simulink model "BLDC_motor_control_v1"  (R2017b)
settings: Solver=FixedStepDiscrete  StartTime=0.0  StopTime=10  FixedStep=1e-5  RelTol=1e-3
values from neighbouring files (symbols this model uses):
  p = 2    [BLDC_model_init.m]
libraries: nesl_utility x41, fl_lib x33, pe_lib x30, simulink x6, pePwmGenerator x2
(part 2 of 2)

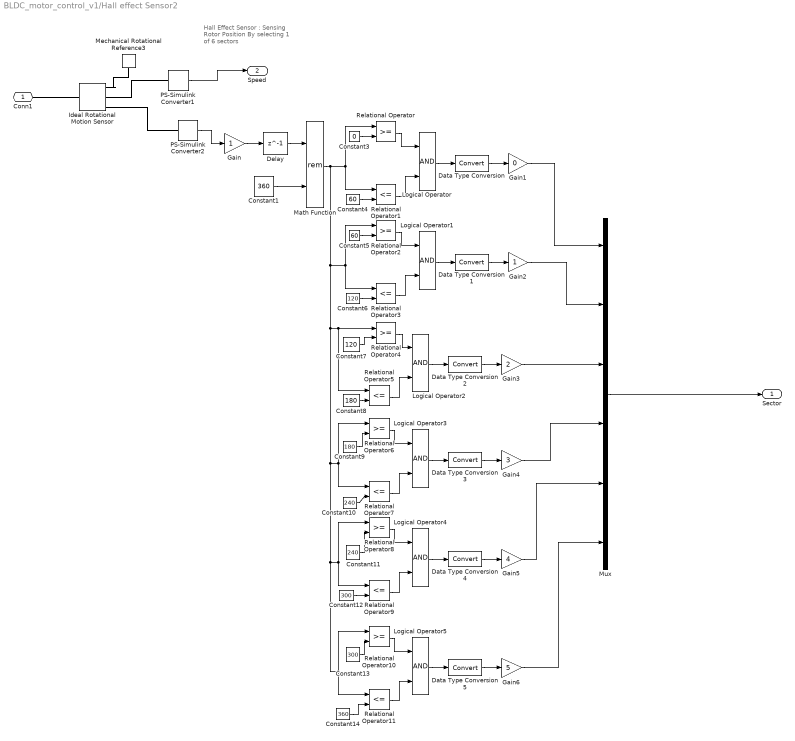
== system BLDC_motor_control_v1/Hall effect Sensor2 ==
  note: Hall Effect Sensor : Sensing Rotor Position By selecting 1 of 6 sectors
  Constant1 : Constant  Value=360
  Constant10 : Constant  Value=240
  Constant11 : Constant  Value=240
  Constant12 : Constant  Value=300
  Constant13 : Constant  Value=300
  Constant14 : Constant  Value=360
  Constant3 : Constant  Value=0
  Constant4 : Constant  Value=60
  Constant5 : Constant  Value=60
  Constant6 : Constant  Value=120
  Constant7 : Constant  Value=120
  Constant8 : Constant  Value=180
  Constant9 : Constant  Value=180
  Data Type Conversion{,1..5} (6 alike) : DataTypeConversion
  Delay : Delay  DelayLength=1
  Gain : Gain
  Gain1 : Gain  Gain=0
  Gain2 : Gain
  Gain3 : Gain  Gain=2
  Gain4 : Gain  Gain=3
  Gain5 : Gain  Gain=4
  Gain6 : Gain  Gain=5
  Ideal Rotational Motion Sensor : fl_lib/Mechanical/Mechanical Sensors/Ideal Rotational Motion Sensor  offset=0 rad
  Logical Operator{,1..5} (6 alike) : Logic  AllPortsSameDT=off  OutDataTypeStr=boolean
  Math Function : Math  Operator=rem  SaturateOnIntegerOverflow=on
  Mechanical Rotational Reference3 : fl_lib/Mechanical/Rotational Elements/Mechanical Rotational Reference
  Mux : Mux  Inputs=6
  PS-Simulink Converter1 : nesl_utility/PS-Simulink Converter  PhysicalDomain=network_engine_domain  SubClassName=ps_output  LeftPortType=input  RightPortType=output  PseudoPeriodic=off  Frequencies=[]  Unit=1  AffineConversion=off
  PS-Simulink Converter2 : nesl_utility/PS-Simulink Converter  PhysicalDomain=network_engine_domain  SubClassName=ps_output  LeftPortType=input  RightPortType=output  PseudoPeriodic=off  Frequencies=[]  Unit=1  AffineConversion=off
  Relational Operator{,2,4,6,8,10} (6 alike) : RelationalOperator  OutDataTypeStr=boolean  RndMeth=Simplest
  Relational Operator{1,3,5,7,9,11} (6 alike) : RelationalOperator  Operator=<=  OutDataTypeStr=boolean  RndMeth=Simplest
  Conn1 : PMIOPort  Port=1  Side=Left
  Sector : Outport
  Speed : Outport  Port=2
  wires:
  PS-Simulink Converter2/1 -> Gain/1
  Gain5/1 -> Mux/5
  Gain/1 -> Delay/1
  Gain6/1 -> Mux/6
  Relational Operator10/1 -> Logical Operator5/1
  Relational Operator6/1 -> Logical Operator3/1
  Data Type Conversion2/1 -> Gain3/1
  Logical Operator/1 -> Data Type Conversion/1
  Constant6/1 -> Relational Operator3/2
  Constant1/1 -> Math Function/2
  Relational Operator5/1 -> Logical Operator2/2
  Relational Operator/1 -> Logical Operator/1
  Relational Operator4/1 -> Logical Operator2/1
  Constant9/1 -> Relational Operator6/2
  Constant10/1 -> Relational Operator7/2
  Mux/1 -> Sector/1
  Constant3/1 -> Relational Operator/2
  Data Type Conversion1/1 -> Gain2/1
  Math Function/1 -> Relational Operator1/1, Relational Operator/1, Relational Operator3/1, Relational Operator2/1, Relational Operator5/1, Relational Operator4/1, Relational Operator11/1, Relational Operator10/1, Relational Operator9/1, Relational Operator8/1, Relational Operator7/1, Relational Operator6/1
  Gain2/1 -> Mux/2
  Constant8/1 -> Relational Operator5/2
  Relational Operator8/1 -> Logical Operator4/1
  Relational Operator2/1 -> Logical Operator1/1
  Gain4/1 -> Mux/4
  Logical Operator1/1 -> Data Type Conversion1/1
  Logical Operator2/1 -> Data Type Conversion2/1
  Gain3/1 -> Mux/3
  Delay/1 -> Math Function/1
  Gain1/1 -> Mux/1
  Logical Operator5/1 -> Data Type Conversion5/1
  Constant14/1 -> Relational Operator11/2
  Constant13/1 -> Relational Operator10/2
  Constant7/1 -> Relational Operator4/2
  Relational Operator11/1 -> Logical Operator5/2
  Data Type Conversion5/1 -> Gain6/1
  Data Type Conversion3/1 -> Gain4/1
  Relational Operator9/1 -> Logical Operator4/2
  Relational Operator7/1 -> Logical Operator3/2
  Relational Operator3/1 -> Logical Operator1/2
  Data Type Conversion/1 -> Gain1/1
  Logical Operator4/1 -> Data Type Conversion4/1
  Data Type Conversion4/1 -> Gain5/1
  Constant5/1 -> Relational Operator2/2
  Constant4/1 -> Relational Operator1/2
  Constant11/1 -> Relational Operator8/2
  PS-Simulink Converter1/1 -> Speed/1
  Logical Operator3/1 -> Data Type Conversion3/1
  Relational Operator1/1 -> Logical Operator/2
  Constant12/1 -> Relational Operator9/2
  connections:
  Ideal Rotational Motion Sensor/RConn3 -- PS-Simulink Converter2/LConn1
  Ideal Rotational Motion Sensor/RConn2 -- PS-Simulink Converter1/LConn1
  Ideal Rotational Motion Sensor/LConn1 -- Conn1/RConn1
  Ideal Rotational Motion Sensor/RConn1 -- Mechanical Rotational Reference3/LConn1

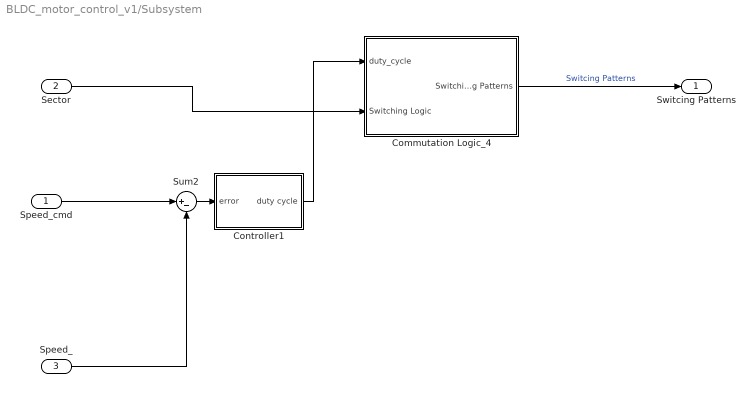
== system BLDC_motor_control_v1/Subsystem ==
  Speed_cmd : Inport  OutDataTypeStr=double  PortDimensions=1  SampleTime=[1.0000000000000001e-05,0]
  Sector : Inport  Port=2  OutDataTypeStr=double  PortDimensions=6  SampleTime=[1.0000000000000001e-05,0]
  Speed_ : Inport  Port=3  OutDataTypeStr=double  PortDimensions=1  SampleTime=[1.0000000000000001e-05,0]
  Commutation Logic_4 : Subsystem
  Controller1 : Subsystem
  Sum2 : Sum  Inputs=|+-
  Switcing Patterns : Outport  OutDataTypeStr=double  PortDimensions=6  SampleTime=[1.0000000000000001e-05,0]
  wires:
  Speed_/1 -> Sum2/2
  Sum2/1 -> Controller1/1(error)
  Controller1/1(duty cycle) -> Commutation Logic_4/1(duty_cycle)
  Commutation Logic_4/1(Switching Patterns) -> Switcing Patterns/1  "Switcing Patterns"
  Speed_cmd/1 -> Sum2/1
  Sector/1 -> Commutation Logic_4/2(Switching Logic)

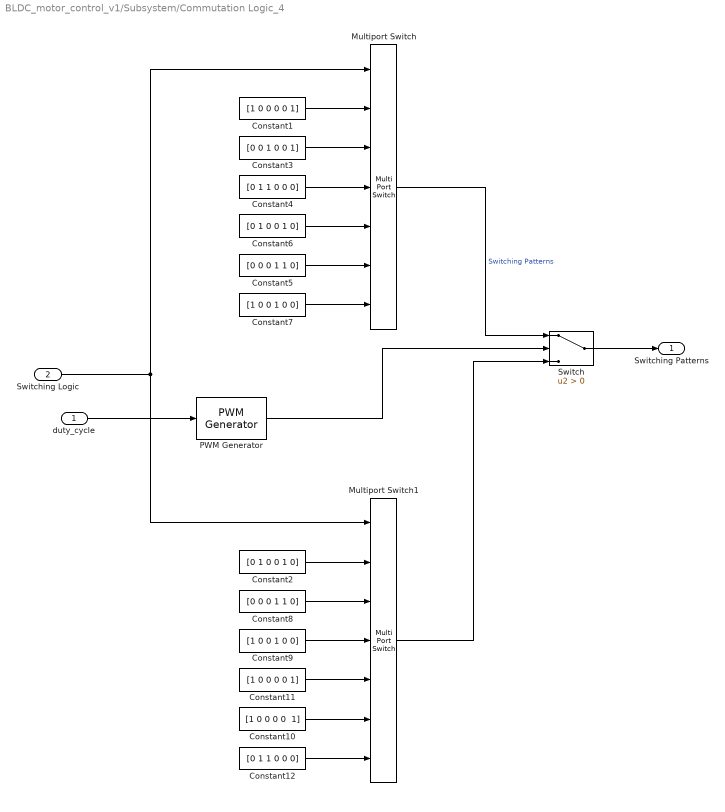
== system BLDC_motor_control_v1/Subsystem/Commutation Logic_4 ==
  duty_cycle : Inport
  Switching Logic : Inport  Port=2
  Constant1 : Constant  Value=[1 0 0 0 0 1]
  Constant10 : Constant  Value="[1 0 0 0 0  1]"
  Constant11 : Constant  Value=[1 0 0 0 0 1]
  Constant12 : Constant  Value=[0 1 1 0 0 0]
  Constant2 : Constant  Value=[0 1 0 0 1 0]
  Constant3 : Constant  Value=[0 0 1 0 0 1]
  Constant4 : Constant  Value=[0 1 1 0 0 0]
  Constant5 : Constant  Value=[0 0 0 1 1 0]
  Constant6 : Constant  Value=[0 1 0 0 1 0]
  Constant7 : Constant  Value=[1 0 0 1 0 0]
  Constant8 : Constant  Value=[0 0 0 1 1 0]
  Constant9 : Constant  Value=[1 0 0 1 0 0]
  Multiport Switch : MultiPortSwitch  DataPortOrder=Zero-based contiguous  Inputs=6
  Multiport Switch1 : MultiPortSwitch  DataPortOrder=Zero-based contiguous  Inputs=6
  PWM Generator : pePwmGenerator/PWM Generator  CarrCount=Up  Tper=0.001  Ts=5e-5
  Switch : Switch  Criteria=u2 > Threshold
  Switching Patterns : Outport
  wires:
  Multiport Switch1/1 -> Switch/3
  Constant11/1 -> Multiport Switch1/5
  Constant10/1 -> Multiport Switch1/6
  Constant2/1 -> Multiport Switch1/2
  Constant8/1 -> Multiport Switch1/3
  Constant9/1 -> Multiport Switch1/4
  Constant12/1 -> Multiport Switch1/7
  Switch/1 -> Switching Patterns/1
  Multiport Switch/1 -> Switch/1  "Switching Patterns"
  PWM Generator/1 -> Switch/2
  duty_cycle/1 -> PWM Generator/1
  Constant5/1 -> Multiport Switch/6
  Constant6/1 -> Multiport Switch/5
  Constant3/1 -> Multiport Switch/3
  Constant7/1 -> Multiport Switch/7
  Constant1/1 -> Multiport Switch/2
  Constant4/1 -> Multiport Switch/4
  Switching Logic/1 -> Multiport Switch/1, Multiport Switch1/1

== system BLDC_motor_control_v1/Subsystem/Controller1 ==
  error : Inport
  PID Controller1 : simulink/Continuous/PID Controller  Controller=PI  TimeDomain=Discrete-time  SampleTime=-1  IntegratorMethod=Forward Euler  FilterMethod=Forward Euler  Form=Parallel  UseFilter=on  ControllerParametersSource=internal  P=0.01  I=5  D=0  N=100  InitialConditionSource=internal  InitialConditionForIntegrator=0  InitialConditionForFilter=0  ExternalReset=none  LimitOutput=off  UpperSaturationLimit=inf  LowerSaturationLimit=-inf  LinearizeAsGain=on  AntiWindupMode=none  Kb=1  TrackingMode=off  Kt=1  PParamMin=[]  PParamMax=[]  IParamMin=[]  IParamMax=[]  DParamMin=[]  DParamMax=[]  NParamMin=[]  NParamMax=[]  KbParamMin=[]  KbParamMax=[]  KtParamMin=[]  KtParamMax=[]  POutMin=[]  POutMax=[]  IOutMin=[]  IOutMax=[]  DOutMin=[]  DOutMax=[]  NOutMin=[]  NOutMax=[]  KbOutMin=[]  KbOutMax=[]  KtOutMin=[]  KtOutMax=[]  IntegratorOutMin=[]  IntegratorOutMax=[]  FilterOutMin=[]  FilterOutMax=[]  SumOutMin=[]  SumOutMax=[]  SumI1OutMin=[]  SumI1OutMax=[]  SumI2OutMin=[]  SumI2OutMax=[]  SumI3OutMin=[]  SumI3OutMax=[]  SumDOutMin=[]  SumDOutMax=[]  SaturationOutMin=[]  SaturationOutMax=[]  IntegratorContinuousStateAttributes=''  IntegratorStateMustResolveToSignalObject=off  IntegratorRTWStateStorageClass=Auto  FilterContinuousStateAttributes=''  FilterStateMustResolveToSignalObject=off  FilterRTWStateStorageClass=Auto  DifferentiatorICPrevScaledInput=0  DifferentiatorOutMin=[]  DifferentiatorOutMax=[]  InitialConditionSetting=State (most efficient)  FilterDiffOutCoefMin=[]  FilterDiffOutCoefMax=[]  SumDenOutMin=[]  SumDenOutMax=[]  SumNumOutMin=[]  SumNumOutMax=[]  ReciprocalOutMin=[]  ReciprocalOutMax=[]  DivideOutMin=[]  DivideOutMax=[]  TunerSelectOption=Transfer Function Based (PID Tuner App)
  duty cycle : Outport
  wires:
  error/1 -> PID Controller1/1
  PID Controller1/1 -> duty cycle/1
